simulink model "satellite_orbit_sim"  (R2025b)
settings: Solver=ode45  StartTime=0.0  StopTime=5676.978028525858  MaxStep=10  RelTol=1e-3
settings Model: Creator=17978  LastModifiedBy=17978

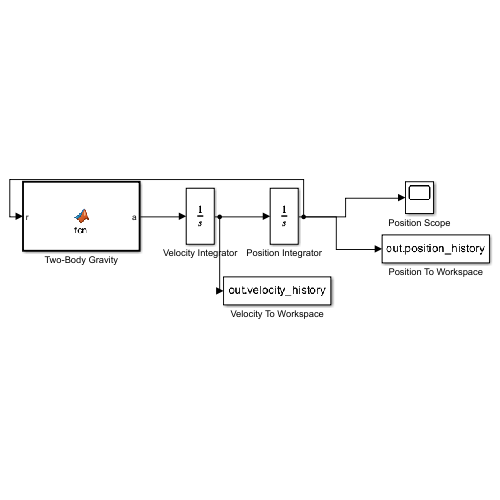
[thumbnail: Simulink's stored preview of the top-level diagram]
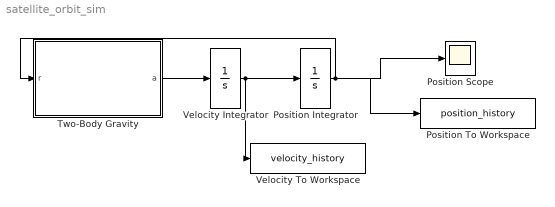
== system satellite_orbit_sim ==
  Position Integrator : Integrator  InitialCondition=[6878.137000000000; 0]
  Position Scope : Scope
  Position To Workspace : ToWorkspace  VariableName=position_history  SaveFormat=Structure With Time  SampleTime=-1
  Two-Body Gravity : MATLAB Function  TreatAsAtomicUnit=on
  Velocity Integrator : Integrator  InitialCondition=[0; 7.612608173224]
  Velocity To Workspace : ToWorkspace  VariableName=velocity_history  SaveFormat=Structure With Time  SampleTime=-1
  wires:
  Two-Body Gravity/1(a) -> Velocity Integrator/1
  Velocity Integrator/1 -> Position Integrator/1, Velocity To Workspace/1
  Position Integrator/1 -> Two-Body Gravity/1(r), Position Scope/1, Position To Workspace/1

== matlab function satellite_orbit_sim/Two-Body Gravity ==
  data: r input; a output
function a = fcn(r)
% Two-body orbital acceleration in the orbital plane.
mu = 398600.4417999999714;
norm_r = sqrt(r(1)^2 + r(2)^2);
a = -mu .* r ./ (norm_r^3);
end
